simulink model "sampleModel201"  (R2021b)
settings: Solver=VariableStepAuto  StartTime=0.0  StopTime=10.0  RelTol=1e-3
libraries: simulink x5
settings Model: Creator=user  LastModifiedBy=user

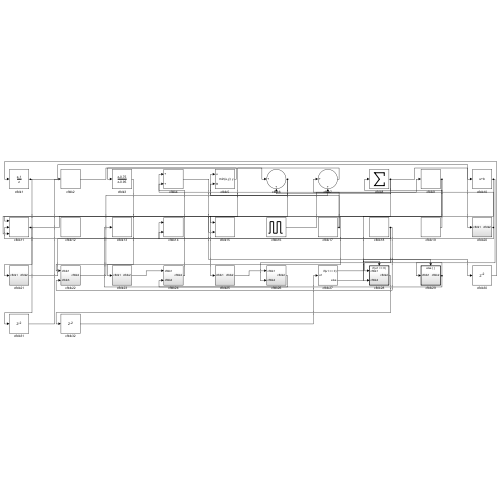
[thumbnail: Simulink's stored preview of the top-level diagram]
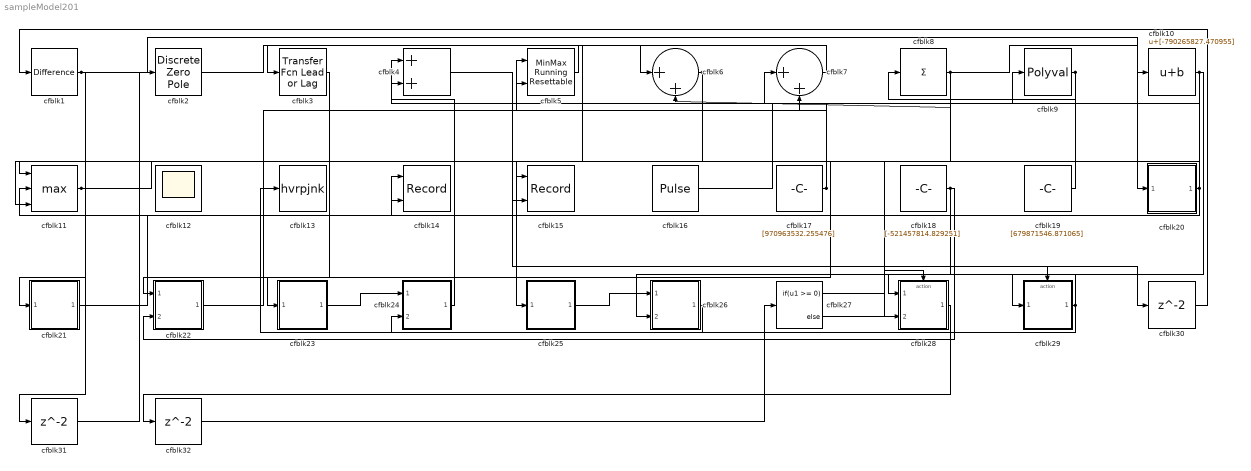
== system sampleModel201 ==
  cfblk1 : simulink/Discrete/Difference  ICPrevInput=0.0  OutMin=[]  OutMax=[]  OutDataTypeStr=Inherit: Inherit via back propagation  OutDataType=fixdt(1, 16)  OutScaling=2^-10  DoSatur=off
  cfblk10 : Bias  Bias=[-790265827.470955]
  cfblk11 : MinMax  Function=max  Inputs=3
  cfblk12 : Scope
      settings: Floating=on
  cfblk13 : ToWorkspace  VariableName=hvrpjnk  SaveFormat=Timeseries  SampleTime=-1
  cfblk14 : Record  FileSettingsInternal="{\"entries\":[{\"content\":{\"excelSettings\":{\"content\":{},\"type\":\"Streamout.ExcelSettings\"}},\"type\":\"Streamout.FileSettingStorage\",\"uuid\":\"5194d8ca-deb6-4edd-b001-44b51bd05890\"}],\"packageUris\":[\"http://schema.mathworks.com/mf0/streamout_blocks/R2020a\"],\"version\":\"1.0\"}"  Layout=[1 1]  SignalsInternal="{\"entries\":[{\"content\":{\"signals\":[{\"content\":{\"blockPath\":[\"sampleModel201/cfblk14\"],\"channel\":[],\"dimensions\":[1],\"domain\":\"sampleModel201/cfblk14\",\"lineColor\":\"#a2142f\",\"plots\":[1],\"port\":1,\"sid\":[\"\"],\"signalID\":7685,\"signalName\":\"cfblk21\"},\"type\":\"RecordBlkView.Signal\",\"uuid\":\"b1914e17-5de9-4d07-bd4e-10ac7d4d30b7\"},{\"content\":{\"blockPath\":[\"sampleModel201/cfblk14\"],\"channel\":[],\"dimensions\":[1],\"domain\":\"sampleModel201/cfblk14\",\"lineColor\":\"#139fff\",\"plots\":[1],\"port\":2,\"sid\":[\"\"],\"signalID\":7689,\"signalName\":\"cfblk20\"},\"type\":\"RecordBlkView.Signal\",\"uuid\":\"2d60233f-8f4c-4c8f-8fc8-0bc09b5b7c69\"}]},\"type\":\"RecordBlkView.InputSignals\",\"uuid\":\"047ee044-3f29-46a5-8b99-54f38227e97f\"}],\"packageUris\":[\"http://schema.mathworks.com/mf0/streamout_blocks/R2020a\"],\"version\":\"1.0\"}"  VisualizationBindings="{\"xyplotplugin\":{\"info\":[{\"series\":[{\"bindingParametersList\":[{\"parameter\":\"X-Axis\",\"signalID\":7685,\"signalName\":\"cfblk21\"},{\"parameter\":\"Y-Axis\",\"signalID\":7689,\"signalName\":\"cfblk20\"}],\"seriesID\":39296}],\"subplotID\":1}]}}"  CompatibilityTag=XY
  cfblk15 : Record  FileSettingsInternal="{\"entries\":[{\"content\":{\"excelSettings\":{\"content\":{},\"type\":\"Streamout.ExcelSettings\"}},\"type\":\"Streamout.FileSettingStorage\",\"uuid\":\"312659b0-d3c8-4785-8936-697f5d01142d\"}],\"packageUris\":[\"http://schema.mathworks.com/mf0/streamout_blocks/R2020a\"],\"version\":\"1.0\"}"  Layout=[1 1]  SignalsInternal="{\"entries\":[{\"content\":{\"signals\":[{\"content\":{\"blockPath\":[\"sampleModel201/cfblk15\"],\"channel\":[],\"dimensions\":[1],\"domain\":\"sampleModel201/cfblk15\",\"lineColor\":\"#a2142f\",\"plots\":[1],\"port\":1,\"sid\":[\"\"],\"signalID\":7693,\"signalName\":\"cfblk11\"},\"type\":\"RecordBlkView.Signal\",\"uuid\":\"acdee433-706e-43ae-995f-6c743a2ff393\"},{\"content\":{\"blockPath\":[\"sampleModel201/cfblk15\"],\"channel\":[],\"dimensions\":[1],\"domain\":\"sampleModel201/cfblk15\",\"lineColor\":\"#139fff\",\"plots\":[1],\"port\":2,\"sid\":[\"\"],\"signalID\":7697,\"signalName\":\"cfblk10\"},\"type\":\"RecordBlkView.Signal\",\"uuid\":\"fdc86f2a-493e-40ff-b875-b66aee590f37\"}]},\"type\":\"RecordBlkView.InputSignals\",\"uuid\":\"98ba482b-33d4-438d-872f-160a207b0858\"}],\"packageUris\":[\"http://schema.mathworks.com/mf0/streamout_blocks/R2020a\"],\"version\":\"1.0\"}"  VisualizationBindings="{\"xyplotplugin\":{\"info\":[{\"series\":[{\"bindingParametersList\":[{\"parameter\":\"X-Axis\",\"signalID\":7693,\"signalName\":\"cfblk11\"},{\"parameter\":\"Y-Axis\",\"signalID\":7697,\"signalName\":\"cfblk10\"}],\"seriesID\":23501}],\"subplotID\":1}]}}"  CompatibilityTag=XY
  cfblk16 : DiscretePulseGenerator  PulseType=Time based  Amplitude=[-839947818.489038]  Period=[47133683.636986]  PulseWidth=5  PhaseDelay=[5.000000]
  cfblk17 : Constant  Value=[970963532.255476]  SampleTime=1
  cfblk18 : Constant  Value=[-521457814.829251]  SampleTime=1
  cfblk19 : Constant  Value=[679871546.871065]  SampleTime=1
  cfblk2 : DiscreteZeroPole  Poles=[0 0.5]  Gain=1
  cfblk20 : Subsystem
  cfblk21 : Subsystem
  cfblk22 : Subsystem
  cfblk23 : Subsystem
  cfblk24 : Subsystem
  cfblk25 : Subsystem
  cfblk26 : Subsystem
  cfblk27 : If  IfExpression=u1 >= 0  SampleTime=1
  cfblk28 : Subsystem  TreatAsAtomicUnit=on
  cfblk29 : Subsystem  TreatAsAtomicUnit=on
  cfblk3 : simulink/Discrete/Transfer Fcn Lead or Lag  PoleZ=0.95  ZeroZ=0.75  ICPrevOutput=0.0  ICPrevInput=0.0  DoSatur=off
      settings: SourceProductBaseCode=SL
  cfblk30 : Delay  SampleTime=1
  cfblk31 : Delay  SampleTime=1
  cfblk32 : Delay  SampleTime=1
  cfblk4 : Sum
  cfblk5 : simulink/Math Operations/MinMax Running Resettable  Function=min  vinit=0.0
  cfblk6 : Sum  Inputs=|++
  cfblk7 : Sum  Inputs=|++
  cfblk8 : Sum  Inputs=+
  cfblk9 : Polyval  Coefs=[ +2.081618890e-019, -1.441693666e-014, +4.719686976e-010, -8.536869453e-006, +1.621573104e-001, -8.087801117e+001 ]
  wires:
  cfblk17/1 -> cfblk7/1, cfblk5/1
  cfblk5/1 -> cfblk3/1
  cfblk9/1 -> cfblk23/1(cfblk1), cfblk11/3
  cfblk7/1 -> cfblk11/1
  cfblk1/1 -> cfblk20/1(cfblk1), cfblk21/1(cfblk1)
  cfblk26/1(cfblk2) -> cfblk13/1
  cfblk21/1(cfblk2) -> cfblk14/1
  cfblk24/1(cfblk2) -> cfblk4/1
  cfblk25/1(cfblk2) -> cfblk26/1(cfblk1)
  cfblk23/1(cfblk2) -> cfblk24/1(cfblk1)
  cfblk10/1 -> cfblk29/1(cfblk1), cfblk15/2
  cfblk20/1(cfblk2) -> cfblk4/2, cfblk14/2
  cfblk2/1 -> cfblk6/1
  cfblk16/1 -> cfblk9/1
  cfblk8/1 -> cfblk6/2, cfblk10/1, cfblk28/2(cfblk4)
  cfblk22/1(cfblk2) -> cfblk7/2
  cfblk3/1 -> cfblk22/1(cfblk1)
  cfblk18/1 -> cfblk22/2(cfblk3), cfblk26/2(cfblk4), cfblk11/2
  cfblk11/1 -> cfblk15/1, cfblk31/1
  cfblk29/1(cfblk2) -> cfblk28/1(cfblk1), cfblk24/2(cfblk4)
  cfblk19/1 -> cfblk8/1
  cfblk6/1 -> cfblk25/1(cfblk1), cfblk5/2
  cfblk27/1 -> cfblk28/Action
  cfblk27/2 -> cfblk29/Action
  cfblk4/1 -> cfblk30/1
  cfblk30/1 -> cfblk1/1
  cfblk31/1 -> cfblk2/1
  cfblk28/1(cfblk2) -> cfblk32/1
  cfblk32/1 -> cfblk27/1

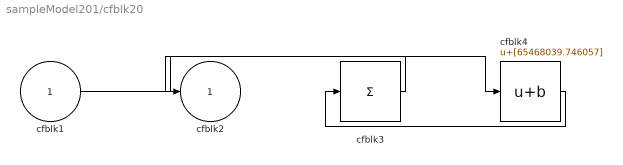
== system sampleModel201/cfblk20 ==
  cfblk1 : Inport
  cfblk3 : Sum  Inputs=+
  cfblk4 : Bias  Bias=[65468039.746057]
  cfblk2 : Outport
  wires:
  cfblk1/1 -> cfblk4/1
  cfblk4/1 -> cfblk3/1
  cfblk3/1 -> cfblk2/1

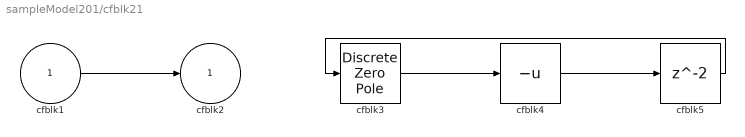
== system sampleModel201/cfblk21 ==
  cfblk1 : Inport
  cfblk3 : DiscreteZeroPole  Poles=[0 0.5]  Gain=1
  cfblk4 : UnaryMinus
  cfblk5 : Delay  SampleTime=1
  cfblk2 : Outport
  wires:
  cfblk3/1 -> cfblk4/1
  cfblk1/1 -> cfblk2/1
  cfblk4/1 -> cfblk5/1
  cfblk5/1 -> cfblk3/1

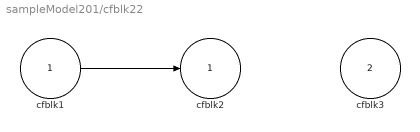
== system sampleModel201/cfblk22 ==
  cfblk1 : Inport
  cfblk3 : Inport  Port=2
  cfblk2 : Outport
  wires:
  cfblk1/1 -> cfblk2/1

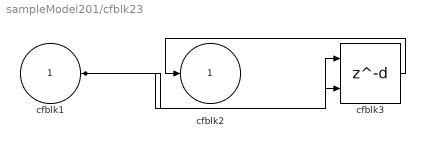
== system sampleModel201/cfblk23 ==
  cfblk1 : Inport
  cfblk3 : Delay  DelayLengthSource=Input port  SampleTime=1
      settings: InputPortMap=u0,p1
  cfblk2 : Outport
  wires:
  cfblk3/1 -> cfblk2/1
  cfblk1/1 -> cfblk3/1, cfblk3/2

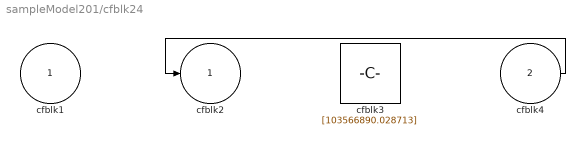
== system sampleModel201/cfblk24 ==
  cfblk1 : Inport
  cfblk4 : Inport  Port=2
  cfblk3 : Constant  Value=[103566890.028713]  SampleTime=1
  cfblk2 : Outport
  wires:
  cfblk4/1 -> cfblk2/1

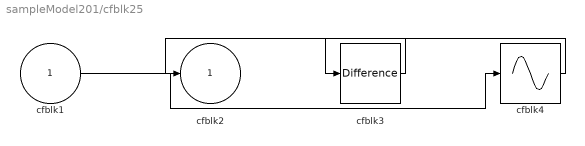
== system sampleModel201/cfblk25 ==
  cfblk1 : Inport
  cfblk3 : simulink/Discrete/Difference  ICPrevInput=0.0  OutMin=[]  OutMax=[]  OutDataTypeStr=Inherit: Inherit via back propagation  OutDataType=fixdt(1, 16)  OutScaling=2^-10  DoSatur=off
  cfblk4 : Sin  TimeSource=Use external signal  SampleTime=0
  cfblk2 : Outport
  wires:
  cfblk4/1 -> cfblk3/1
  cfblk1/1 -> cfblk4/1
  cfblk3/1 -> cfblk2/1

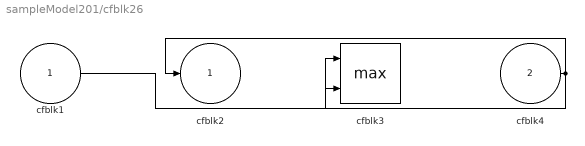
== system sampleModel201/cfblk26 ==
  cfblk1 : Inport
  cfblk4 : Inport  Port=2
  cfblk3 : MinMax  Function=max  Inputs=2
  cfblk2 : Outport
  wires:
  cfblk4/1 -> cfblk2/1, cfblk3/2
  cfblk1/1 -> cfblk3/1

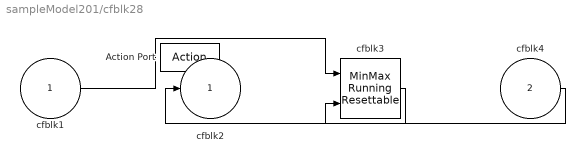
== system sampleModel201/cfblk28 ==
  cfblk1 : Inport
  cfblk4 : Inport  Port=2
  Action Port : ActionPort  ActionPortLabel=if(u1 >= 0)
  cfblk3 : simulink/Math Operations/MinMax Running Resettable  Function=min  vinit=0.0
  cfblk2 : Outport
  wires:
  cfblk3/1 -> cfblk2/1
  cfblk1/1 -> cfblk3/1
  cfblk4/1 -> cfblk3/2

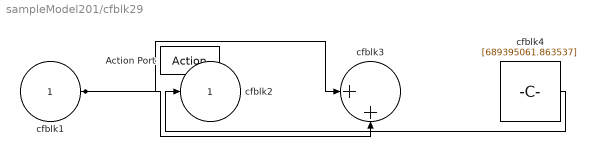
== system sampleModel201/cfblk29 ==
  cfblk1 : Inport
  Action Port : ActionPort  ActionPortLabel=else
  cfblk3 : Sum  Inputs=|++
  cfblk4 : Constant  Value=[689395061.863537]  SampleTime=1
  cfblk2 : Outport
  wires:
  cfblk4/1 -> cfblk2/1
  cfblk1/1 -> cfblk3/1, cfblk3/2
